simulink model "Controller"  (R2024a)
settings: Solver=FixedStepDiscrete  StartTime=0.0  StopTime=inf  FixedStep=Ts  RelTol=1e-3
undefined symbols (not defined in the file or in its folder): DiscIntNeverNeededParam, OmegaVector, T, Ts, U0, Wr0
libraries: DRC_SimulinkLibrary x6, simulink x2, slpidlib x2
settings Model: Creator=evansolingen  LastModifiedBy=glazzerini
settings SolverCC: AlgebraicLoopSolver=TrustRegion
settings DataIOCC: LimitDataPoints=on  SaveFormat=Array  SignalLoggingSaveFormat=ModelDataLogs  SaveOutput=off  SignalLogging=off  SaveTime=off  ReturnWorkspaceOutputs=off
settings OptimizationCC: ExpressionDepthLimit=2147483647  LifeSpan=inf
settings DebuggingCC: MergeDetectMultiDrivingBlocksExec=none  SolverPrmCheckMsg=warning  MultiTaskDSMMsg=warning  MultiTaskCondExecSysMsg=none  FcnCallInpInsideContextMsg=warning  UnconnectedInputMsg=warning  UnconnectedOutputMsg=warning  UnconnectedLineMsg=warning  AllowSymbolicDim=off  StateNameClashWarn=warning  SFUnexpectedBacktrackingDiag=warning  SFNoUnconditionalDefaultTransitionDiag=warning  SFExecutionAtInitializationDiag=none  ArithmeticOperatorsInVariantConditions=warning
settings HardwareCC: ProdBitPerPointer=32  ProdBitPerSizeT=32  ProdBitPerPtrDiffT=32  ProdLargestAtomicFloat=None  ProdIntDivRoundTo=Undefined  ProdEndianess=Unspecified  ProdWordSize=32  ProdHWDeviceType=32-bit Generic
settings ModelReferenceCC: UpdateModelReferenceTargets=Force  EnableRefExpFcnMdlSchedulingChecks=on  PropagateSignalLabelsOutOfModel=off
settings SFSimCC: SimUseLocalCustomCode=off  SimParseCustomCode=off  CustomCodeUndefinedFunction=UseInterfaceOnly
settings RTWCC: Description=DISCON DLL Target (for use with GH BLADED)  SystemTargetFile=discon.tlc  TemplateMakefile=discon_vc.tmf  RTWUseLocalCustomCode=off  GPUComputeCapability=3.5  DLArmComputeVersion=19.05
settings CodeAppCC: StateflowObjectComments=on
settings GRTTargetCC: TargetLangStandard=C89/C90 (ANSI)  CombineOutputUpdateFcns=off  GRTInterface=on  UseToolchainInfoCompliant=off  ExtModeMexFile=noextcomm
settings ConfigComp: CovMetricSettings=dw  CovSaveCumulativeToWorkspaceVar=on  CovSaveSingleToWorkspaceVar=on  CovExternalEMLEnable=off

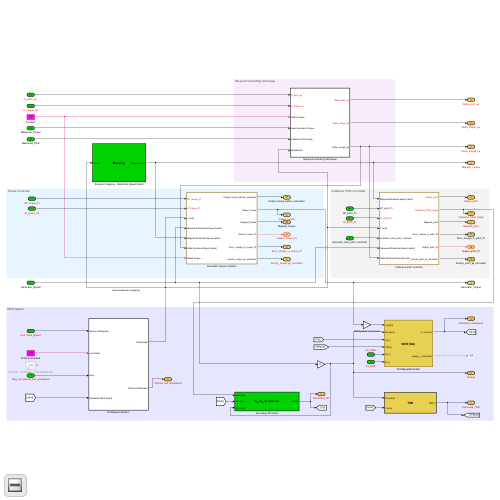
[thumbnail: Simulink's stored preview of the top-level diagram]
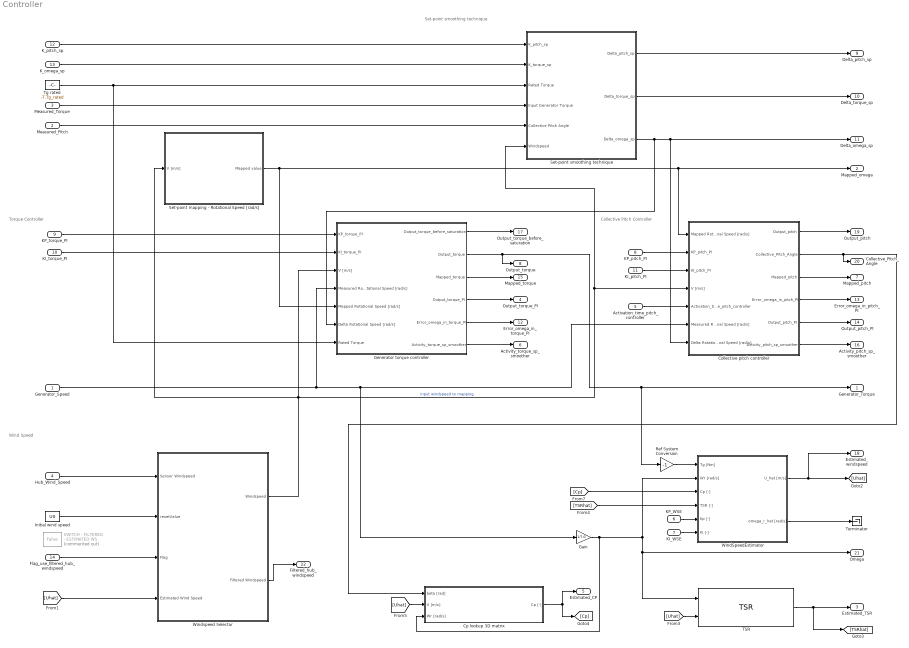
== system Controller ==
  note: Wind Speed
  note: Collective Pitch Controller
  note: Torque Controller
  note: Set-point smoothing technique
  Generator_Speed : Inport
  Measured_Pitch : Inport  Port=2  PortDimensions=1
  Measured_Torque : Inport  Port=3  PortDimensions=1
  Hub_Wind_Speed : Inport  Port=4  PortDimensions=1
  Activation_time_pitch_controller : Inport  Port=5  PortDimensions=1
  KP_WSE : Inport  Port=6  PortDimensions=1
  KI_WSE : Inport  Port=7  PortDimensions=1
  KP_pitch_PI : Inport  Port=8  PortDimensions=1
  KP_torque_PI : Inport  Port=9  PortDimensions=1
  KI_torque_PI : Inport  Port=10  PortDimensions=1
  KI_pitch_PI : Inport  Port=11  PortDimensions=1
  K_pitch_sp : Inport  Port=12  PortDimensions=1
  K_omega_sp : Inport  Port=13  PortDimensions=1
  Flag_use_filtered_hub_windspeed : Inport  Port=14  PortDimensions=1
  Collective pitch controller : Subsystem
  Cp lookup 3D matrix : Subsystem  AncestorBlock=DRC_SimulinkLibrary/Cpqt lookup  mask(Coefficient look-up){CpqtGrid=T.Cp, PitchVector=deg2rad(T.CPitch), WindSpeedVector=T.CWindSpeed, OmegaVector=T.COmega}
      mask prompts: CpqtGrid "Cp/Cq/Ct grid [-]"; PitchVector "Pitch vector [rad]"; WindSpeedVector "Wind Speed vector [m/s]"; OmegaVector "Omega vector [rad/s]"
      mask help: Coefficient look-up matrices for power coefficient (Cp), torque coefficient (Cq), and thrust coefficient (Ct). The Pitch, Wind-speed and Omega data should be 1-dimensional vectors of sizes p, q and r respectively. The provided coefficient matrix should be of size p x q x r.
      mask Display: disp('{\bf\fontsize{12}C_p, C_q, C_t look-up}', 'texmode', 'on');
  Gain : Gain  Gain=1/T.G
  Generator torque controller : Subsystem
  Initial wind speed : Constant  Value=U0
  Ref System Conversion : Gain  Gain=-1
  SWITCH - FILTERED - ESTIMATED WS : Constant  Commented=on  Value=false
  Set-point mapping - Rotational Speed [rad/s] : Subsystem  AncestorBlock=DRC_SimulinkLibrary/Set-point mapping  mask(Mapping look-up){MappingVector=T.OmegaFB, WindSpeedVector=T.WindSpeedFF}
      mask help: Mapping look-up for rotational speed or collective pitch angle vs windspeed. The input data should be a 1-dimensional value. The provided value will represent the mapping.
      mask Display: disp('{\bf\fontsize{12}Mapping}', 'texmode', 'on');
  Set-point smoothing technique : Subsystem
  TSR : DRC_SimulinkLibrary/TSR  RotorRadius=T.R
  Terminator : Terminator
  "Tg rated " : Constant  Value=-T.Tg_rated
  WindSpeedEstimator : Subsystem  AncestorBlock=DRC_SimulinkLibrary/WindSpeedEstimator  mask(Wind speed estimator (I&I)){R=T.R, Tr_max=T.Tr_max, G=T.G, JLss=T.Jlss, rho=T.rho, omega_r_0=Wr0, V0=U0, Ts=Ts}
      mask prompts: R "Rotor radius [m]"; Tr_max "Max. exp. rotor torque [Nm]"; G "Gearbox ratio"; JLss "Drivetrain inertia (LSS)"; rho "Air density [kg/m^3]"; omega_r_0 "Rotor speed initial condition"; V0 "Wind speed initial condition"; Ts "Sampling time [s]"
      mask help: Immersion and Invariance (I&I) wind speed estimator. Uses prior power coefficient information of the turbine to obtain an estimate of the aerodynamic rotor torque. Together with the measured generator torque and rotor speed, an estimate of the wind speed is computed.
      mask Display: disp('{\bf\fontsize{12}WSE (I&I)}', 'texmode', 'on');
  Windspeed Selector : Subsystem
  Generator_Torque : Outport
  Mapped_omega : Outport  Port=2  PortDimensions=1
  Estimated_TSR : Outport  Port=3  PortDimensions=1
  Output_torque_PI : Outport  Port=4  PortDimensions=1
  Estimated_CP : Outport  Port=5  PortDimensions=1
  Activity_torque_sp_smoother : Outport  Port=6  PortDimensions=1
  Mapped_pitch : Outport  Port=7  PortDimensions=1
  Output_torque : Outport  Port=8  PortDimensions=1
  Delta_pitch_sp : Outport  Port=9  PortDimensions=1
  Delta_torque_sp : Outport  Port=10  PortDimensions=1
  Delta_omega_sp : Outport  Port=11  PortDimensions=1
  Error_omega_in_torque_PI : Outport  Port=12  PortDimensions=1
  Error_omega_in_pitch_PI : Outport  Port=13  PortDimensions=1
  Output_pitch_PI : Outport  Port=14  PortDimensions=1
  Mapped_torque : Outport  Port=15  PortDimensions=1
  Activity_pitch_sp_smoother : Outport  Port=16  PortDimensions=1
  Output_torque_before_saturation : Outport  Port=17  PortDimensions=1
  Estimated_windspeed : Outport  Port=18  PortDimensions=1
  Output_pitch : Outport  Port=19  PortDimensions=1
  Collective_Pitch_Angle : Outport  Port=20  PortDimensions=1
  Omega : Outport  Port=21  PortDimensions=1
  Filtered_hub_windspeed : Outport  Port=22  PortDimensions=1
  wires:
  K_omega_sp/1 -> Set-point smoothing technique/2(K_torque_sp)
  Activation_time_pitch_controller/1 -> Collective pitch controller/5(Activation_time_pitch_controller)
  Generator torque controller/1(Output_torque_before_saturation) -> Output_torque_before_saturation/1
  KP_torque_PI/1 -> Generator torque controller/1(KP_torque_PI)
  "Tg rated "/1 -> Generator torque controller/7(Rated Torque), Set-point smoothing technique/3(Rated Torque)
  K_pitch_sp/1 -> Set-point smoothing technique/1(K_pitch_sp)
  Set-point smoothing technique/3(Delta_omega_sp) -> Generator torque controller/6(Delta Rotational Speed [rad/s]), Collective pitch controller/7(Delta Rotational Speed [rad/s]), Delta_omega_sp/1
  KI_torque_PI/1 -> Generator torque controller/2(KI_torque_PI)
  Set-point smoothing technique/2(Delta_torque_sp) -> Delta_torque_sp/1
  Set-point smoothing technique/1(Delta_pitch_sp) -> Delta_pitch_sp/1
  Set-point mapping - Rotational Speed [rad/s]/1(Mapped value) -> Generator torque controller/5(Mapped Rotational Speed [rad/s]), Collective pitch controller/1(Mapped Rotational Speed [rad/s]), Mapped_omega/1
  Collective pitch controller/3(Mapped_pitch) -> Mapped_pitch/1
  Measured_Torque/1 -> Set-point smoothing technique/4(Input Generator Torque)
  KP_pitch_PI/1 -> Collective pitch controller/2(KP_pitch_PI)
  Measured_Pitch/1 -> Set-point smoothing technique/5(Collective Pitch Angle)
  Generator torque controller/3(Mapped_torque) -> Mapped_torque/1
  KI_pitch_PI/1 -> Collective pitch controller/3(KI_pitch_PI)
  Collective pitch controller/1(Output_pitch) -> Output_pitch/1
  Generator torque controller/4(Output_torque_PI) -> Output_torque_PI/1
  Generator torque controller/5(Error_omega_in_torque_PI) -> Error_omega_in_torque_PI/1
  Collective pitch controller/4(Error_omega_in_pitch_PI) -> Error_omega_in_pitch_PI/1
  Collective pitch controller/5(Output_pitch_PI) -> Output_pitch_PI/1
  Collective pitch controller/6(Activity_pitch_sp_smoother) -> Activity_pitch_sp_smoother/1
  Generator torque controller/6(Activity_torque_sp_smoother) -> Activity_torque_sp_smoother/1
  WindSpeedEstimator/1(U_hat [m/s]) -> Estimated_windspeed/1, [Uhat]
  Cp lookup 3D matrix/1(Cp [-]) -> Estimated_CP/1, [Cp]
  TSR/1 -> [TSRhat], Estimated_TSR/1
  WindSpeedEstimator/2(omega_r_hat [rad/s]) -> Terminator/1
  Gain/1 -> TSR/1, Omega/1, WindSpeedEstimator/2(Wr [rad/s]), Cp lookup 3D matrix/3(Wr [rad/s])
  Windspeed Selector/1(Windspeed) -> Set-point mapping - Rotational Speed [rad/s]/1(V [m/s]), Generator torque controller/3(V [m/s]), Collective pitch controller/4(V [m/s]), Set-point smoothing technique/6(Windspeed)  "input windspeed to mapping"
  Hub_Wind_Speed/1 -> Windspeed Selector/1(Sensor Windspeed)
  Initial wind speed/1 -> Windspeed Selector/2(resetValue)
  Flag_use_filtered_hub_windspeed/1 -> Windspeed Selector/3(Flag)
  [Uhat] -> Windspeed Selector/4(Estimated Wind Speed)
  Windspeed Selector/2(Filtered Windspeed) -> Filtered_hub_windspeed/1
  Collective pitch controller/2(Collective_Pitch_Angle) -> Cp lookup 3D matrix/1(beta [rad]), Collective_Pitch_Angle/1
  Generator torque controller/2(Output_torque) -> Ref System Conversion/1, Generator_Torque/1, Output_torque/1
  Generator_Speed/1 -> Generator torque controller/4(Measured Rotational Speed [rad/s]), Collective pitch controller/6(Measured Rotational Speed [rad/s]), Gain/1
  KP_WSE/1 -> WindSpeedEstimator/5(Kp [-])
  KI_WSE/1 -> WindSpeedEstimator/6(Ki [-])
  [Uhat] -> Cp lookup 3D matrix/2(V [m/s])
  [TSRhat] -> WindSpeedEstimator/4(TSR [-])
  [Uhat] -> TSR/2
  [Cp] -> WindSpeedEstimator/3(Cp [-])
  Ref System Conversion/1 -> WindSpeedEstimator/1(Tg [Nm])

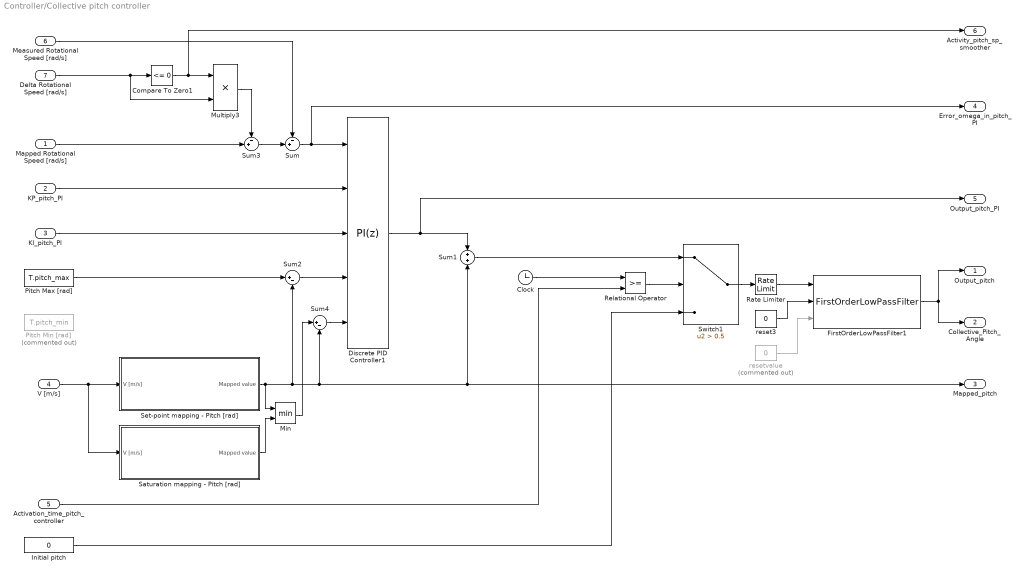
== system Controller/Collective pitch controller ==
  Mapped Rotational Speed [rad/s] : Inport
  KP_pitch_PI : Inport  Port=2  PortDimensions=1
  KI_pitch_PI : Inport  Port=3  PortDimensions=1
  V [m/s] : Inport  Port=4
  Activation_time_pitch_controller : Inport  Port=5  PortDimensions=1
  Measured Rotational Speed [rad/s] : Inport  Port=6
  Delta Rotational Speed [rad/s] : Inport  Port=7
  Clock : Clock
  Compare To Zero1 : simulink/Logic and Bit Operations/Compare To Zero  relop=<=  OutDataTypeStr=boolean
  Discrete PID Controller1 : slpidlib/PID Controller  Controller=PI  Form=Parallel  TimeDomain=Discrete-time  UseExternalTs=off  SampleTime=-1  IntegratorMethod=Forward Euler  FilterMethod=Forward Euler  ControllerParametersSource=external  P=1  I=1  UseKiTs=off  D=0  UseExternalDerivativeSource=off  N=100  UseFilter=on  TunerSelectOption=Transfer Function Based (PID Tuner App)  InitialConditionSource=internal  InitialConditionForIntegrator=0  InitialConditionForFilter=0  DifferentiatorICPrevScaledInput=0  ExternalReset=none  TrackingMode=off  Kt=1  LimitOutput=on  SatLimitsSource=external  UpperSaturationLimit=inf  LowerSaturationLimit=-inf  LinearizeAsGain=off  AntiWindupMode=clamping  Kb=1  LimitIntegrator=off  UpperIntegratorSaturationLimit=inf  LowerIntegratorSaturationLimit=-inf  POutMin=[]  POutMax=[]  IOutMin=[]  IOutMax=[]  DOutMin=[]  DOutMax=[]  NOutMin=[]  NOutMax=[]  SumOutMin=[]  SumOutMax=[]  SaturationOutMin=[]  SaturationOutMax=[]  PParamMin=[]  PParamMax=[]  IParamMin=[]  IParamMax=[]  DParamMin=[]  DParamMax=[]  NParamMin=[]  NParamMax=[]  KbParamMin=[]  KbParamMax=[]  KtParamMin=[]  KtParamMax=[]  KbOutMin=[]  KbOutMax=[]  KtOutMin=[]  KtOutMax=[]  IntegratorOutMin=[]  IntegratorOutMax=[]  FilterOutMin=[]  FilterOutMax=[]  SumI1OutMin=[]  SumI1OutMax=[]  SumI2OutMin=[]  SumI2OutMax=[]  SumI3OutMin=[]  SumI3OutMax=[]  SumI4OutMin=[]  SumI4OutMax=[]  SumDOutMin=[]  SumDOutMax=[]  DifferentiatorOutMin=[]  DifferentiatorOutMax=[]  FilterDiffOutCoefMin=[]  FilterDiffOutCoefMax=[]  ReciprocalOutMin=[]  ReciprocalOutMax=[]  SumDenOutMin=[]  SumDenOutMax=[]  SumNumOutMin=[]  SumNumOutMax=[]  DivideOutMin=[]  DivideOutMax=[]  UdiffTsProdOutMin=[]  UdiffTsProdOutMax=[]  NTsProdOutMin=[]  NTsProdOutMax=[]  UintegralTsProdOutMin=[]  UintegralTsProdOutMax=[]  UngainTsProdOutMin=[]  UngainTsProdOutMax=[]  ClampingZeroOutDataTypeStr=Inherit: Inherit via back propagation  ClampingZeroOutMin=[]  ClampingZeroOutMax=[]  FilterDenConstantOutDataTypeStr=Inherit: Inherit via back propagation  FilterDenConstantOutMin=[]  FilterDenConstantOutMax=[]  PCopyOutDataTypeStr=Inherit: Inherit via back propagation  PCopyOutMin=[]  PCopyOutMax=[]  NCopyOutDataTypeStr=Inherit: Inherit via back propagation  NCopyOutMin=[]  NCopyOutMax=[]  IntegratorContinuousStateAttributes=''  IntegratorStateMustResolveToSignalObject=off  IntegratorRTWStateStorageClass=Auto  FilterContinuousStateAttributes=''  FilterStateMustResolveToSignalObject=off  FilterRTWStateStorageClass=Auto  ParallelPVariant=ExternalParameters  IdealPVariant=Disabled  IVariant=ExternalParameters  DVariant=Disabled  IntegratorVariant=Discrete  SatVariant=External  AWVariant=DiscClampingParallel  PCopyVariant=Disabled  TRVariant=Disabled  FdbkBlocksVariant=Forward  IdealPFdbkVariant=Disabled  SatFdbkVariant=Disabled  DerivativeFilterVariant=Disabled  NVariant=Disabled  NCopyVariant=Disabled_SignalSpec  FilterICVariant=Disabled  IntegratorICVariant=InternalICs  ExternalResetVariant=Disabled  TRSumVariant=Passthrough  SumFdbkVariant=Disabled  SumVariant=Sum_PI  TsampFilterVariant=InternalTs  TsampNgainVariant=Passthrough  TsampIntegralVariant=Disabled_SignalSpec  ExternalSaturationOutDataTypeStr=Inherit: Same as second input  DerivativeSourceVariant=Disabled
      settings: LibrarySourceBlock=simulink/Discrete/Discrete PID Controller
  FirstOrderLowPassFilter1 : DRC_SimulinkLibrary/FirstOrderLowPassFilter  wc=3.14  Ts=0.01
  Initial pitch : Constant  Value=0
  Min : MinMax  Inputs=2
  Multiply3 : Product
  Pitch Max [rad] : Constant  Value=T.pitch_max
  Pitch Min [rad] : Constant  Commented=on  Value=T.pitch_min
  Rate Limiter : RateLimiter  RisingSlewLimit=T.pitch_max_rate  FallingSlewLimit=T.pitch_min_rate  SampleTimeMode=inherited
  Relational Operator : RelationalOperator  OutDataTypeStr=boolean  RndMeth=Simplest  InputSameDT=off
  Saturation mapping - Pitch [rad] : Subsystem  AncestorBlock=DRC_SimulinkLibrary/Set-point mapping  mask(Mapping look-up){MappingVector=T.PitchSatMap, WindSpeedVector=T.WindSpeedSatMap}
      mask help: Mapping look-up for rotational speed or collective pitch angle vs windspeed. The input data should be a 1-dimensional value. The provided value will represent the mapping.
      mask Display: disp('{\bf\fontsize{12}Mapping}', 'texmode', 'on');
  Set-point mapping - Pitch [rad] : Subsystem  AncestorBlock=DRC_SimulinkLibrary/Set-point mapping  mask(Mapping look-up){MappingVector=T.PitchFF, WindSpeedVector=T.WindSpeedFF}
      mask help: Mapping look-up for rotational speed or collective pitch angle vs windspeed. The input data should be a 1-dimensional value. The provided value will represent the mapping.
      mask Display: disp('{\bf\fontsize{12}Mapping}', 'texmode', 'on');
  Sum : Sum  Inputs=-+|
  Sum1 : Sum  Inputs=+|+
  Sum2 : Sum  Inputs=|+-
  Sum3 : Sum  Inputs=-+|
  Sum4 : Sum  Inputs=|+-
  Switch1 : Switch  Criteria=u2 > Threshold  Threshold=0.5  SaturateOnIntegerOverflow=off  InputSameDT=off
  reset3 : Constant  Value=0
  resetvalue : Constant  Commented=on  Value=0
  Output_pitch : Outport  PortDimensions=1
  Collective_Pitch_Angle : Outport  Port=2  PortDimensions=1
  Mapped_pitch : Outport  Port=3
  Error_omega_in_pitch_PI : Outport  Port=4
  Output_pitch_PI : Outport  Port=5
  Activity_pitch_sp_smoother : Outport  Port=6
  wires:
  KP_pitch_PI/1 -> Discrete PID Controller1/2
  Set-point mapping - Pitch [rad]/1(Mapped value) -> Min/1, Sum4/2, Mapped_pitch/1, Sum1/2, Sum2/2
  Sum/1 -> Error_omega_in_pitch_PI/1, Discrete PID Controller1/1
  KI_pitch_PI/1 -> Discrete PID Controller1/3
  V [m/s]/1 -> Set-point mapping - Pitch [rad]/1(V [m/s]), Saturation mapping - Pitch [rad]/1(V [m/s])
  Discrete PID Controller1/1 -> Sum1/1, Output_pitch_PI/1
  Measured Rotational Speed [rad/s]/1 -> Sum/1
  Clock/1 -> Relational Operator/1
  Activation_time_pitch_controller/1 -> Relational Operator/2
  Relational Operator/1 -> Switch1/2
  Initial pitch/1 -> Switch1/3
  Switch1/1 -> Rate Limiter/1
  Multiply3/1 -> Sum3/1
  Mapped Rotational Speed [rad/s]/1 -> Sum3/2
  Sum3/1 -> Sum/2
  Delta Rotational Speed [rad/s]/1 -> Multiply3/2, Compare To Zero1/1
  reset3/1 -> FirstOrderLowPassFilter1/2
  resetvalue/1 -> FirstOrderLowPassFilter1/3
  Compare To Zero1/1 -> Activity_pitch_sp_smoother/1, Multiply3/1
  Sum1/1 -> Switch1/1
  Pitch Max [rad]/1 -> Sum2/1
  Sum2/1 -> Discrete PID Controller1/4
  Sum4/1 -> Discrete PID Controller1/5
  Saturation mapping - Pitch [rad]/1(Mapped value) -> Min/2
  Rate Limiter/1 -> FirstOrderLowPassFilter1/1
  FirstOrderLowPassFilter1/1 -> Output_pitch/1, Collective_Pitch_Angle/1
  Min/1 -> Sum4/1

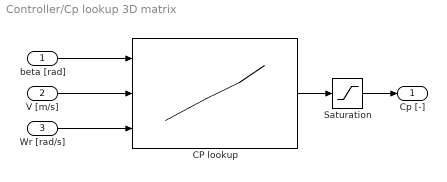
== system Controller/Cp lookup 3D matrix ==
  beta [rad] : Inport
  V [m/s] : Inport  Port=2
  Wr [rad/s] : Inport  Port=3
  CP lookup : Lookup_n-D  NumberOfTableDimensions=3  BreakpointsForDimension1=PitchVector  BreakpointsForDimension2=WindSpeedVector  BreakpointsForDimension3=OmegaVector  Table=CpqtGrid  InternalRulePriority=Speed  RndMeth=Simplest
      settings: InputPortMap=u0,u1,u2
  Saturation : Saturate  UpperLimit=1.0  LowerLimit=eps
  Cp [-] : Outport
  wires:
  Saturation/1 -> Cp [-]/1
  CP lookup/1 -> Saturation/1
  V [m/s]/1 -> CP lookup/2
  Wr [rad/s]/1 -> CP lookup/3
  beta [rad]/1 -> CP lookup/1

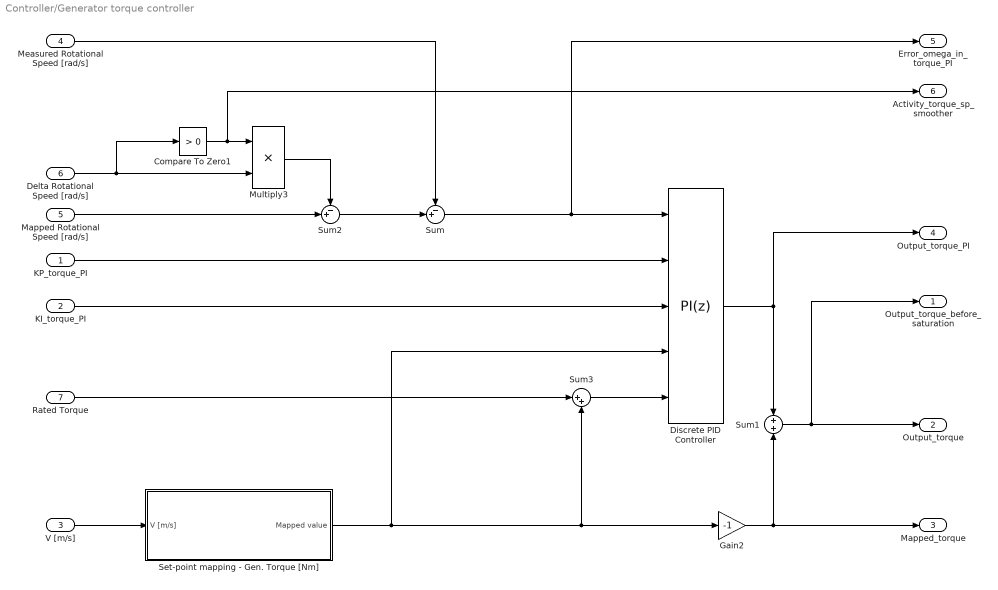
== system Controller/Generator torque controller ==
  KP_torque_PI : Inport  PortDimensions=1
  KI_torque_PI : Inport  Port=2  PortDimensions=1
  V [m/s] : Inport  Port=3
  Measured Rotational Speed [rad/s] : Inport  Port=4
  Mapped Rotational Speed [rad/s] : Inport  Port=5
  Delta Rotational Speed [rad/s] : Inport  Port=6
  Rated Torque : Inport  Port=7
  Compare To Zero1 : simulink/Logic and Bit Operations/Compare To Zero  relop=>  OutDataTypeStr=boolean
  Discrete PID Controller : slpidlib/PID Controller  Controller=PI  Form=Parallel  TimeDomain=Discrete-time  UseExternalTs=off  SampleTime=-1  IntegratorMethod=Forward Euler  FilterMethod=Forward Euler  ControllerParametersSource=external  P=1  I=1  UseKiTs=off  D=0  UseExternalDerivativeSource=off  N=100  UseFilter=on  TunerSelectOption=Transfer Function Based (PID Tuner App)  InitialConditionSource=internal  InitialConditionForIntegrator=0  InitialConditionForFilter=0  DifferentiatorICPrevScaledInput=0  ExternalReset=none  TrackingMode=off  Kt=1  LimitOutput=on  SatLimitsSource=external  UpperSaturationLimit=0  LowerSaturationLimit=-inf  LinearizeAsGain=off  AntiWindupMode=clamping  Kb=1  LimitIntegrator=off  UpperIntegratorSaturationLimit=inf  LowerIntegratorSaturationLimit=-inf  POutMin=[]  POutMax=[]  IOutMin=[]  IOutMax=[]  DOutMin=[]  DOutMax=[]  NOutMin=[]  NOutMax=[]  SumOutMin=[]  SumOutMax=[]  SaturationOutMin=[]  SaturationOutMax=[]  PParamMin=[]  PParamMax=[]  IParamMin=[]  IParamMax=[]  DParamMin=[]  DParamMax=[]  NParamMin=[]  NParamMax=[]  KbParamMin=[]  KbParamMax=[]  KtParamMin=[]  KtParamMax=[]  KbOutMin=[]  KbOutMax=[]  KtOutMin=[]  KtOutMax=[]  IntegratorOutMin=[]  IntegratorOutMax=[]  FilterOutMin=[]  FilterOutMax=[]  SumI1OutMin=[]  SumI1OutMax=[]  SumI2OutMin=[]  SumI2OutMax=[]  SumI3OutMin=[]  SumI3OutMax=[]  SumI4OutMin=[]  SumI4OutMax=[]  SumDOutMin=[]  SumDOutMax=[]  DifferentiatorOutMin=[]  DifferentiatorOutMax=[]  FilterDiffOutCoefMin=[]  FilterDiffOutCoefMax=[]  ReciprocalOutMin=[]  ReciprocalOutMax=[]  SumDenOutMin=[]  SumDenOutMax=[]  SumNumOutMin=[]  SumNumOutMax=[]  DivideOutMin=[]  DivideOutMax=[]  UdiffTsProdOutMin=[]  UdiffTsProdOutMax=[]  NTsProdOutMin=[]  NTsProdOutMax=[]  UintegralTsProdOutMin=[]  UintegralTsProdOutMax=[]  UngainTsProdOutMin=[]  UngainTsProdOutMax=[]  ClampingZeroOutDataTypeStr=Inherit: Inherit via back propagation  ClampingZeroOutMin=[]  ClampingZeroOutMax=[]  FilterDenConstantOutDataTypeStr=Inherit: Inherit via back propagation  FilterDenConstantOutMin=[]  FilterDenConstantOutMax=[]  PCopyOutDataTypeStr=Inherit: Inherit via back propagation  PCopyOutMin=[]  PCopyOutMax=[]  NCopyOutDataTypeStr=Inherit: Inherit via back propagation  NCopyOutMin=[]  NCopyOutMax=[]  IntegratorContinuousStateAttributes=''  IntegratorStateMustResolveToSignalObject=off  IntegratorRTWStateStorageClass=Auto  FilterContinuousStateAttributes=''  FilterStateMustResolveToSignalObject=off  FilterRTWStateStorageClass=Auto  ParallelPVariant=ExternalParameters  IdealPVariant=Disabled  IVariant=ExternalParameters  DVariant=Disabled  IntegratorVariant=Discrete  SatVariant=External  AWVariant=DiscClampingParallel  PCopyVariant=Disabled  TRVariant=Disabled  FdbkBlocksVariant=Forward  IdealPFdbkVariant=Disabled  SatFdbkVariant=Disabled  DerivativeFilterVariant=Disabled  NVariant=Disabled  NCopyVariant=Disabled_SignalSpec  FilterICVariant=Disabled  IntegratorICVariant=InternalICs  ExternalResetVariant=Disabled  TRSumVariant=Passthrough  SumFdbkVariant=Disabled  SumVariant=Sum_PI  TsampFilterVariant=InternalTs  TsampNgainVariant=Passthrough  TsampIntegralVariant=Disabled_SignalSpec  ExternalSaturationOutDataTypeStr=Inherit: Same as second input  DerivativeSourceVariant=Disabled
      settings: LibrarySourceBlock=simulink/Discrete/Discrete PID Controller
  Gain2 : Gain  Gain=-1
  Multiply3 : Product
  Set-point mapping - Gen. Torque [Nm] : Subsystem  AncestorBlock=DRC_SimulinkLibrary/Set-point mapping  mask(Mapping look-up){MappingVector=T.GenTorqueFF, WindSpeedVector=T.WindSpeedFF}
      mask help: Mapping look-up for rotational speed or collective pitch angle vs windspeed. The input data should be a 1-dimensional value. The provided value will represent the mapping.
      mask Display: disp('{\bf\fontsize{12}Mapping}', 'texmode', 'on');
  Sum : Sum  Inputs=-+|
  Sum1 : Sum  Inputs=+|+
  Sum2 : Sum  Inputs=-+|
  Sum3 : Sum  Inputs=|++
  Output_torque_before_saturation : Outport  PortDimensions=1
  Output_torque : Outport  Port=2
  Mapped_torque : Outport  Port=3  PortDimensions=1
  Output_torque_PI : Outport  Port=4
  Error_omega_in_torque_PI : Outport  Port=5
  Activity_torque_sp_smoother : Outport  Port=6
  wires:
  Discrete PID Controller/1 -> Sum1/1, Output_torque_PI/1
  KP_torque_PI/1 -> Discrete PID Controller/2
  KI_torque_PI/1 -> Discrete PID Controller/3
  V [m/s]/1 -> Set-point mapping - Gen. Torque [Nm]/1(V [m/s])
  Set-point mapping - Gen. Torque [Nm]/1(Mapped value) -> Gain2/1, Sum3/2, Discrete PID Controller/4
  Sum/1 -> Error_omega_in_torque_PI/1, Discrete PID Controller/1
  Measured Rotational Speed [rad/s]/1 -> Sum/1
  Delta Rotational Speed [rad/s]/1 -> Multiply3/2, Compare To Zero1/1
  Multiply3/1 -> Sum2/1
  Mapped Rotational Speed [rad/s]/1 -> Sum2/2
  Sum2/1 -> Sum/2
  Sum1/1 -> Output_torque/1, Output_torque_before_saturation/1
  Compare To Zero1/1 -> Multiply3/1, Activity_torque_sp_smoother/1
  Gain2/1 -> Mapped_torque/1, Sum1/2
  Rated Torque/1 -> Sum3/1
  Sum3/1 -> Discrete PID Controller/5

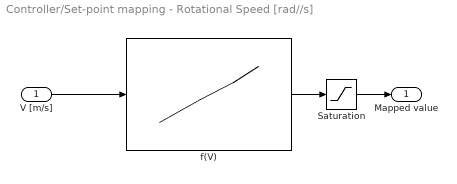
== system Controller/Set-point mapping - Rotational Speed [rad//s] ==
  V [m/s] : Inport
  Saturation : Saturate  UpperLimit=max(T.GenTorqueFF)  LowerLimit=0
  f(V) : Lookup_n-D  NumberOfTableDimensions=1  BreakpointsForDimension1=WindSpeedVector  BreakpointsForDimension2=WindSpeedVector  BreakpointsForDimension3=OmegaVector  Table=MappingVector  InternalRulePriority=Speed  RndMeth=Simplest
  Mapped value : Outport
  wires:
  V [m/s]/1 -> f(V)/1
  f(V)/1 -> Saturation/1
  Saturation/1 -> Mapped value/1

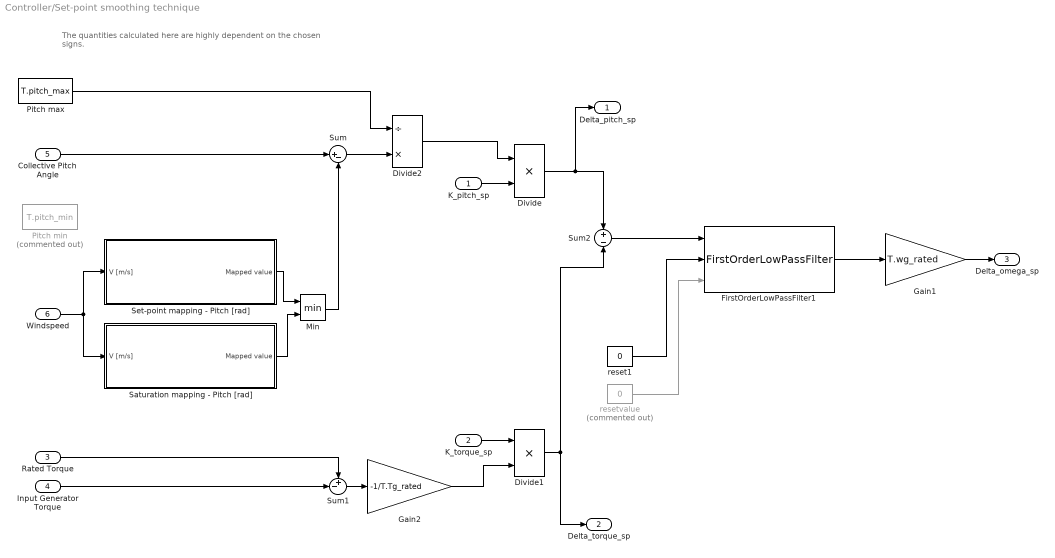
== system Controller/Set-point smoothing technique ==
  note: The quantities calculated here are highly dependent on the chosen signs.
  K_pitch_sp : Inport  PortDimensions=1
  K_torque_sp : Inport  Port=2  PortDimensions=1
  Rated Torque : Inport  Port=3
  Input Generator Torque : Inport  Port=4
  Collective Pitch Angle : Inport  Port=5
  Windspeed : Inport  Port=6
  Divide : Product  Inputs=**
  Divide1 : Product  Inputs=**
  Divide2 : Product  Inputs=/*
  FirstOrderLowPassFilter1 : DRC_SimulinkLibrary/FirstOrderLowPassFilter  wc=0.628  Ts=0.01
  Gain1 : Gain  Gain=T.wg_rated
  Gain2 : Gain  Gain=-1/T.Tg_rated
  Min : MinMax  Inputs=2
  Pitch max : Constant  Value=T.pitch_max
  Pitch min : Constant  Commented=on  Value=T.pitch_min
  Saturation mapping - Pitch [rad] : Subsystem  AncestorBlock=DRC_SimulinkLibrary/Set-point mapping  mask(Mapping look-up){MappingVector=T.PitchSatMap, WindSpeedVector=T.WindSpeedSatMap}
      mask help: Mapping look-up for rotational speed or collective pitch angle vs windspeed. The input data should be a 1-dimensional value. The provided value will represent the mapping.
      mask Display: disp('{\bf\fontsize{12}Mapping}', 'texmode', 'on');
  Set-point mapping - Pitch [rad] : Subsystem  AncestorBlock=DRC_SimulinkLibrary/Set-point mapping  mask(Mapping look-up){MappingVector=T.PitchFF, WindSpeedVector=T.WindSpeedFF}
      mask help: Mapping look-up for rotational speed or collective pitch angle vs windspeed. The input data should be a 1-dimensional value. The provided value will represent the mapping.
      mask Display: disp('{\bf\fontsize{12}Mapping}', 'texmode', 'on');
  Sum : Sum  Inputs=|+-
  Sum1 : Sum  Inputs=+-|
  Sum2 : Sum  Inputs=+|-
  reset1 : Constant  Value=0
  resetvalue : Constant  Commented=on  Value=0
  Delta_pitch_sp : Outport  PortDimensions=1
  Delta_torque_sp : Outport  Port=2  PortDimensions=1
  Delta_omega_sp : Outport  Port=3
  wires:
  Pitch max/1 -> Divide2/1
  Collective Pitch Angle/1 -> Sum/1
  Rated Torque/1 -> Sum1/1
  Sum1/1 -> Gain2/1
  Input Generator Torque/1 -> Sum1/2
  Divide1/1 -> Sum2/2, Delta_torque_sp/1
  Divide2/1 -> Divide/1
  K_pitch_sp/1 -> Divide/2
  K_torque_sp/1 -> Divide1/1
  Gain2/1 -> Divide1/2
  Divide/1 -> Sum2/1, Delta_pitch_sp/1
  Sum2/1 -> FirstOrderLowPassFilter1/1
  reset1/1 -> FirstOrderLowPassFilter1/2
  resetvalue/1 -> FirstOrderLowPassFilter1/3
  FirstOrderLowPassFilter1/1 -> Gain1/1
  Gain1/1 -> Delta_omega_sp/1
  Sum/1 -> Divide2/2
  Set-point mapping - Pitch [rad]/1(Mapped value) -> Min/1
  Windspeed/1 -> Saturation mapping - Pitch [rad]/1(V [m/s]), Set-point mapping - Pitch [rad]/1(V [m/s])
  Saturation mapping - Pitch [rad]/1(Mapped value) -> Min/2
  Min/1 -> Sum/2

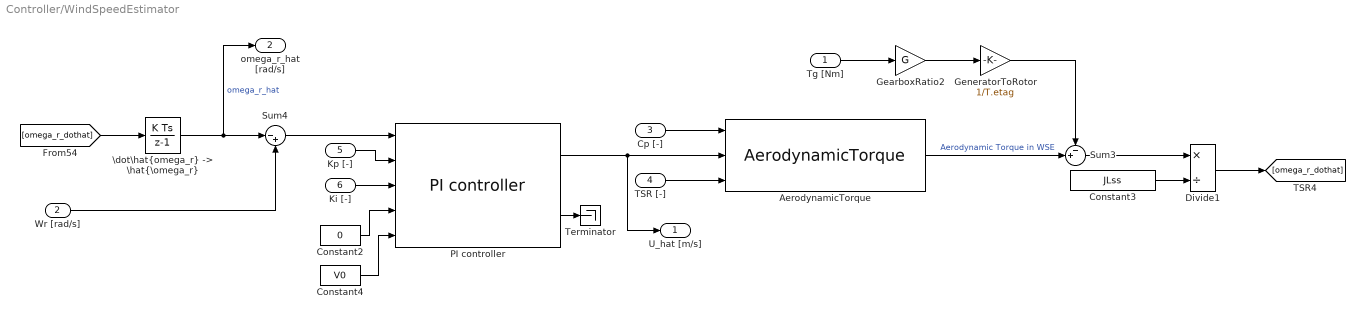
== system Controller/WindSpeedEstimator ==
  Tg [Nm] : Inport
  Wr [rad/s] : Inport  Port=2
  Cp [-] : Inport  Port=3
  TSR [-] : Inport  Port=4
  Kp [-] : Inport  Port=5
  Ki [-] : Inport  Port=6
  AerodynamicTorque : DRC_SimulinkLibrary/AerodynamicTorque  R=R  rho=rho  TrMax=Tr_max
  Constant2 : Constant  Value=0
  Constant3 : Constant  Value=JLss
  Constant4 : Constant  Value=V0
  Divide1 : Product  Inputs=*/
  GearboxRatio2 : Gain  Gain=G
  GeneratorToRotor : Gain  Gain=1/T.etag
  PI controller : DRC_SimulinkLibrary/PI controller  minSatValue=-inf  maxSatValue=inf  Ts=Ts
  Sum3 : Sum  Inputs=-+|
  Sum4 : Sum  Inputs=|-+
  Terminator : Terminator
  "\\dot\\hat{omega_r} -> \\hat{\\omega_r}" : DiscreteIntegrator  InitialCondition=omega_r_0  SampleTime=Ts  ICPrevOutput=DiscIntNeverNeededParam  ICPrevScaledInput=DiscIntNeverNeededParam
  U_hat [m/s] : Outport
  omega_r_hat [rad/s] : Outport  Port=2
  wires:
  PI controller/2 -> Terminator/1
  Constant4/1 -> PI controller/5
  Constant2/1 -> PI controller/4
  Ki [-]/1 -> PI controller/3
  Kp [-]/1 -> PI controller/2
  Sum4/1 -> PI controller/1
  TSR [-]/1 -> AerodynamicTorque/3
  Cp [-]/1 -> AerodynamicTorque/1
  Wr [rad/s]/1 -> Sum4/2
  Tg [Nm]/1 -> GearboxRatio2/1
  [omega_r_dothat] -> "\\dot\\hat{omega_r} -> \\hat{\\omega_r}"/1
  Sum3/1 -> Divide1/1
  Constant3/1 -> Divide1/2
  GearboxRatio2/1 -> GeneratorToRotor/1
  "\\dot\\hat{omega_r} -> \\hat{\\omega_r}"/1 -> omega_r_hat [rad/s]/1, Sum4/1  "omega_r_hat"
  AerodynamicTorque/1 -> Sum3/2  "Aerodynamic Torque in WSE"
  Divide1/1 -> [omega_r_dothat]
  PI controller/1 -> AerodynamicTorque/2, U_hat [m/s]/1
  GeneratorToRotor/1 -> Sum3/1

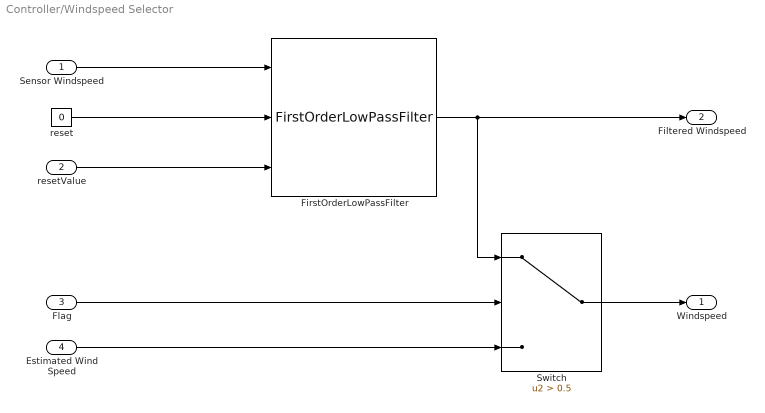
== system Controller/Windspeed Selector ==
  Sensor Windspeed : Inport
  resetValue : Inport  Port=2
  Flag : Inport  Port=3
  Estimated Wind Speed : Inport  Port=4
  FirstOrderLowPassFilter : DRC_SimulinkLibrary/FirstOrderLowPassFilter  wc=3.14  Ts=0.01
  Switch : Switch  Criteria=u2 > Threshold  Threshold=0.5  SaturateOnIntegerOverflow=off  InputSameDT=off
  reset : Constant  Value=0
  Windspeed : Outport
  Filtered Windspeed : Outport  Port=2
  wires:
  resetValue/1 -> FirstOrderLowPassFilter/3
  FirstOrderLowPassFilter/1 -> Filtered Windspeed/1, Switch/1
  Flag/1 -> Switch/2
  Estimated Wind Speed/1 -> Switch/3
  Sensor Windspeed/1 -> FirstOrderLowPassFilter/1
  reset/1 -> FirstOrderLowPassFilter/2
  Switch/1 -> Windspeed/1

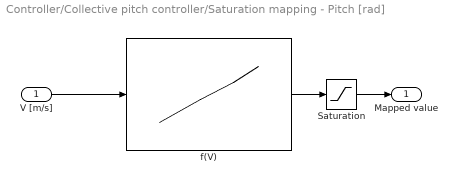
== system Controller/Collective pitch controller/Saturation mapping - Pitch [rad] ==
  V [m/s] : Inport
  Saturation : Saturate  UpperLimit=max(T.PitchFF)  LowerLimit=min(T.PitchFF)
  f(V) : Lookup_n-D  NumberOfTableDimensions=1  BreakpointsForDimension1=WindSpeedVector  BreakpointsForDimension2=WindSpeedVector  BreakpointsForDimension3=OmegaVector  Table=MappingVector  InternalRulePriority=Speed  RndMeth=Simplest
  Mapped value : Outport
  wires:
  V [m/s]/1 -> f(V)/1
  f(V)/1 -> Saturation/1
  Saturation/1 -> Mapped value/1

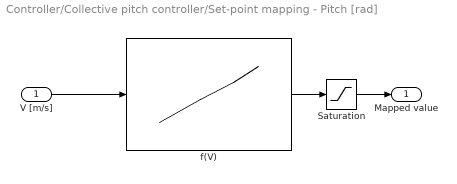
== system Controller/Collective pitch controller/Set-point mapping - Pitch [rad] ==
  V [m/s] : Inport
  Saturation : Saturate  UpperLimit=max(T.PitchFF)  LowerLimit=min(T.PitchFF)
  f(V) : Lookup_n-D  NumberOfTableDimensions=1  BreakpointsForDimension1=WindSpeedVector  BreakpointsForDimension2=WindSpeedVector  BreakpointsForDimension3=OmegaVector  Table=MappingVector  InternalRulePriority=Speed  RndMeth=Simplest
  Mapped value : Outport
  wires:
  V [m/s]/1 -> f(V)/1
  f(V)/1 -> Saturation/1
  Saturation/1 -> Mapped value/1

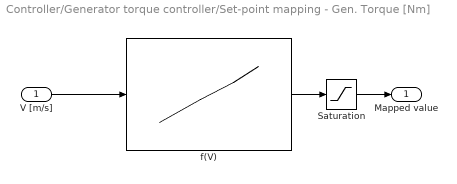
== system Controller/Generator torque controller/Set-point mapping - Gen. Torque [Nm] ==
  V [m/s] : Inport
  Saturation : Saturate  UpperLimit=max(T.GenTorqueFF)  LowerLimit=0
  f(V) : Lookup_n-D  NumberOfTableDimensions=1  BreakpointsForDimension1=WindSpeedVector  BreakpointsForDimension2=WindSpeedVector  BreakpointsForDimension3=OmegaVector  Table=MappingVector  InternalRulePriority=Speed  RndMeth=Simplest
  Mapped value : Outport
  wires:
  V [m/s]/1 -> f(V)/1
  f(V)/1 -> Saturation/1
  Saturation/1 -> Mapped value/1

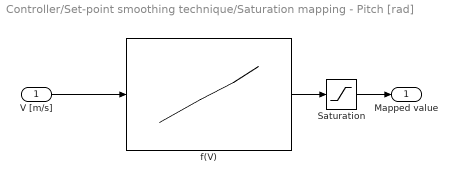
== system Controller/Set-point smoothing technique/Saturation mapping - Pitch [rad] ==
  V [m/s] : Inport
  Saturation : Saturate  UpperLimit=max(T.PitchFF)  LowerLimit=min(T.PitchFF)
  f(V) : Lookup_n-D  NumberOfTableDimensions=1  BreakpointsForDimension1=WindSpeedVector  BreakpointsForDimension2=WindSpeedVector  BreakpointsForDimension3=OmegaVector  Table=MappingVector  InternalRulePriority=Speed  RndMeth=Simplest
  Mapped value : Outport
  wires:
  V [m/s]/1 -> f(V)/1
  f(V)/1 -> Saturation/1
  Saturation/1 -> Mapped value/1

== system Controller/Set-point smoothing technique/Set-point mapping - Pitch [rad] ==
  V [m/s] : Inport
  Saturation : Saturate  UpperLimit=max(T.PitchFF)  LowerLimit=min(T.PitchFF)
  f(V) : Lookup_n-D  NumberOfTableDimensions=1  BreakpointsForDimension1=WindSpeedVector  BreakpointsForDimension2=WindSpeedVector  BreakpointsForDimension3=OmegaVector  Table=MappingVector  InternalRulePriority=Speed  RndMeth=Simplest
  Mapped value : Outport
  wires:
  V [m/s]/1 -> f(V)/1
  f(V)/1 -> Saturation/1
  Saturation/1 -> Mapped value/1
